simulink model "SecRwRtStArmScrnCtrl"  (R2018b)
settings: Solver=FixedStepDiscrete  StartTime=0.0  StopTime=10.0  FixedStep=0.01  RelTol=1e-3
undefined symbols (not defined in the file or in its folder): KeSMSuMdMotFinshdTm_Val, KeSMSuMdRetryTm1_Val, KeSMSuModeReqDurgTm_Val, KeSMSwSecRwRtStArmScrnEnTrigBitMask_Val
libraries: StCtrlLib x1
settings Model: Creator=sn2xws  LastModifiedBy=sn2xws
settings DataIOCC: SaveFormat=StructureWithTime
settings OptimizationCC: DefaultParameterBehavior=Inlined  EnhancedBackFolding=on  PassReuseOutputArgsAs=Individual arguments  ZeroExternalMemoryAtStartup=off  ZeroInternalMemoryAtStartup=off  OptimizeBlockOrder=speed  DifferentSizesBufferReuse=on  OptimizationCustomize=off
settings DebuggingCC: ParameterTunabilityLossMsg=error
settings ModelReferenceCC: ModelReferenceNumInstancesAllowed=Single
settings SFSimCC: MATLABDynamicMemAlloc=off
settings RTWCC: SystemTargetFile=autosar.tlc  GenCodeOnly=on  TemplateMakefile=ert_default_tmf  Description=AUTOSAR  GenerateReport=on  IncludeHyperlinkInReport=on  LaunchReport=on  GenerateTraceInfo=on  GenerateTraceReport=on  GenerateTraceReportSl=on  GenerateTraceReportSf=on  GenerateTraceReportEml=on
settings CodeAppCC: ForceParamTrailComments=on  IgnoreCustomStorageClasses=off  OperatorAnnotations=on  SimulinkDataObjDesc=on  SFDataObjDesc=on  InsertBlockDesc=on
settings STFCustomTargetCC: TargetLangStandard=C99 (ISO)  MultiwordLength=256  ParMdlRefBuildCompliant=on  CompOptLevelCompliant=on  IncludeMdlTerminateFcn=off  CombineOutputUpdateFcns=on  SuppressErrorStatus=on  ERTCustomFileBanners=on  SupportNonFinite=off  SupportComplex=off  SupportContinuousTime=off  SupportNonInlinedSFcns=off  RemoveResetFunc=on  MATLABClassNameForMDSCustomization=Simulink.SoftwareTarget.ERTCustomization  AutosarCompliant=on  UseToolchainInfoCompliant=on  LookupTableObjectStructAxisOrder=2,1,3,4,...  LUTObjectStructOrderEvenSpacing=Size,Table,Breakpoints  SystemTargetFile=autosar.tlc
settings ERTTargetCC: TargetLangStandard=C99 (ISO)  ConcurrentExecutionCompliant=off  IncludeMdlTerminateFcn=off  SuppressErrorStatus=on  SupportNonFinite=off  SupportComplex=off  ModelStepFunctionPrototypeControlCompliant=off  CPPClassGenCompliant=off  AutosarCompliant=on  LookupTableObjectStructAxisOrder=2,1,3,4,...  LUTObjectStructOrderEvenSpacing=Size,Table,Breakpoints  InlinedParameterPlacement=NonHierarchical  ERTCustomFileTemplate=example_file_process.tlc  ERTFilePackagingFormat=Compact

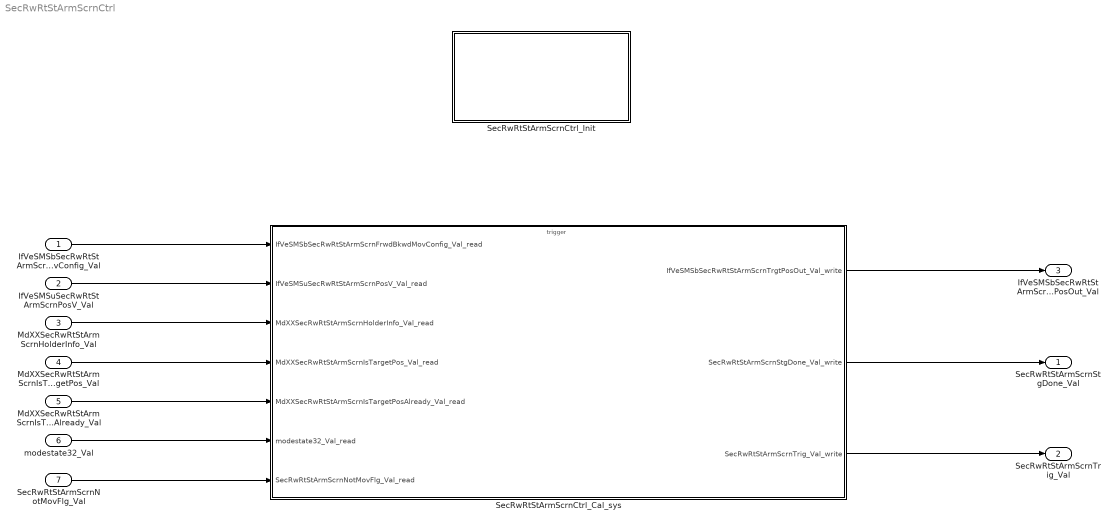
== system SecRwRtStArmScrnCtrl ==
  IfVeSMSbSecRwRtStArmScrnFrwdBkwdMovConfig_Val : Inport  OutDataTypeStr=boolean  PortDimensions=1
  IfVeSMSuSecRwRtStArmScrnPosV_Val : Inport  Port=2  OutDataTypeStr=boolean  PortDimensions=1
  MdXXSecRwRtStArmScrnHolderInfo_Val : Inport  Port=3  OutDataTypeStr=uint32  PortDimensions=1
  MdXXSecRwRtStArmScrnIsTargetPos_Val : Inport  Port=4  OutDataTypeStr=uint32  PortDimensions=1
  MdXXSecRwRtStArmScrnIsTargetPosAlready_Val : Inport  Port=5  OutDataTypeStr=uint32  PortDimensions=1
  modestate32_Val : Inport  Port=6  OutDataTypeStr=uint32  PortDimensions=1
  SecRwRtStArmScrnNotMovFlg_Val : Inport  Port=7  OutDataTypeStr=boolean  PortDimensions=1
  SecRwRtStArmScrnCtrl_Cal_sys : Subsystem
  SecRwRtStArmScrnCtrl_Init : Subsystem
  SecRwRtStArmScrnStgDone_Val : Outport  OutDataTypeStr=boolean  PortDimensions=1
  SecRwRtStArmScrnTrig_Val : Outport  Port=2  OutDataTypeStr=boolean  PortDimensions=1
  IfVeSMSbSecRwRtStArmScrnTrgtPosOut_Val : Outport  Port=3  OutDataTypeStr=boolean  PortDimensions=1
  wires:
  IfVeSMSbSecRwRtStArmScrnFrwdBkwdMovConfig_Val/1 -> SecRwRtStArmScrnCtrl_Cal_sys/1(IfVeSMSbSecRwRtStArmScrnFrwdBkwdMovConfig_Val_read)
  IfVeSMSuSecRwRtStArmScrnPosV_Val/1 -> SecRwRtStArmScrnCtrl_Cal_sys/2(IfVeSMSuSecRwRtStArmScrnPosV_Val_read)
  MdXXSecRwRtStArmScrnHolderInfo_Val/1 -> SecRwRtStArmScrnCtrl_Cal_sys/3(MdXXSecRwRtStArmScrnHolderInfo_Val_read)
  MdXXSecRwRtStArmScrnIsTargetPos_Val/1 -> SecRwRtStArmScrnCtrl_Cal_sys/4(MdXXSecRwRtStArmScrnIsTargetPos_Val_read)
  MdXXSecRwRtStArmScrnIsTargetPosAlready_Val/1 -> SecRwRtStArmScrnCtrl_Cal_sys/5(MdXXSecRwRtStArmScrnIsTargetPosAlready_Val_read)
  modestate32_Val/1 -> SecRwRtStArmScrnCtrl_Cal_sys/6(modestate32_Val_read)
  SecRwRtStArmScrnNotMovFlg_Val/1 -> SecRwRtStArmScrnCtrl_Cal_sys/7(SecRwRtStArmScrnNotMovFlg_Val_read)
  SecRwRtStArmScrnCtrl_Cal_sys/1(IfVeSMSbSecRwRtStArmScrnTrgtPosOut_Val_write) -> IfVeSMSbSecRwRtStArmScrnTrgtPosOut_Val/1
  SecRwRtStArmScrnCtrl_Cal_sys/2(SecRwRtStArmScrnStgDone_Val_write) -> SecRwRtStArmScrnStgDone_Val/1
  SecRwRtStArmScrnCtrl_Cal_sys/3(SecRwRtStArmScrnTrig_Val_write) -> SecRwRtStArmScrnTrig_Val/1

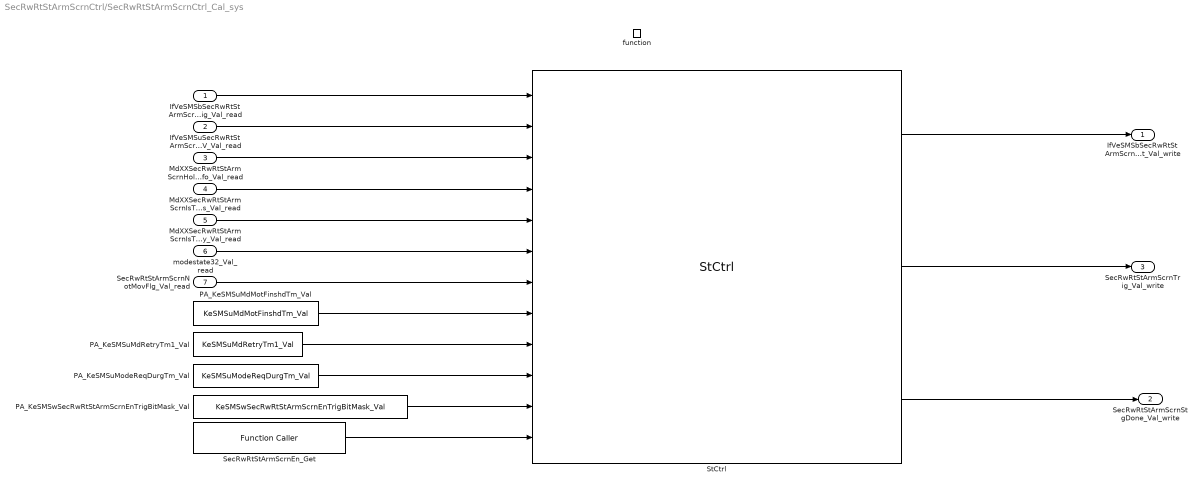
== system SecRwRtStArmScrnCtrl/SecRwRtStArmScrnCtrl_Cal_sys ==
  IfVeSMSbSecRwRtStArmScrnFrwdBkwdMovConfig_Val_read : Inport
  IfVeSMSuSecRwRtStArmScrnPosV_Val_read : Inport  Port=2
  MdXXSecRwRtStArmScrnHolderInfo_Val_read : Inport  Port=3
  MdXXSecRwRtStArmScrnIsTargetPos_Val_read : Inport  Port=4
  MdXXSecRwRtStArmScrnIsTargetPosAlready_Val_read : Inport  Port=5
  modestate32_Val_read : Inport  Port=6
  SecRwRtStArmScrnNotMovFlg_Val_read : Inport  Port=7
  function : TriggerPort  TriggerType=function-call  IsSimulinkFunction=on  FunctionName=SecRwRtStArmScrnCtrl_Cal  VariantControl=(inherit)
  PA_KeSMSuMdMotFinshdTm_Val : Constant  Value=KeSMSuMdMotFinshdTm_Val
  PA_KeSMSuMdRetryTm1_Val : Constant  Value=KeSMSuMdRetryTm1_Val
  PA_KeSMSuModeReqDurgTm_Val : Constant  Value=KeSMSuModeReqDurgTm_Val
  PA_KeSMSwSecRwRtStArmScrnEnTrigBitMask_Val : Constant  Value=KeSMSwSecRwRtStArmScrnEnTrigBitMask_Val
  SecRwRtStArmScrnEn_Get : FunctionCaller  FunctionPrototype=data = SecRwRtStArmScrnEn_Get()  OutputArgumentSpecifications=uint32(1)
  StCtrl : StCtrlLib/StCtrl  SystemSampleTime=-1
  IfVeSMSbSecRwRtStArmScrnTrgtPosOut_Val_write : Outport
      settings: EnsureOutportIsVirtual=on
  SecRwRtStArmScrnStgDone_Val_write : Outport  Port=2
      settings: EnsureOutportIsVirtual=on
  SecRwRtStArmScrnTrig_Val_write : Outport  Port=3
      settings: EnsureOutportIsVirtual=on
  wires:
  StCtrl/3 -> SecRwRtStArmScrnStgDone_Val_write/1
  StCtrl/1 -> IfVeSMSbSecRwRtStArmScrnTrgtPosOut_Val_write/1
  StCtrl/2 -> SecRwRtStArmScrnTrig_Val_write/1
  PA_KeSMSwSecRwRtStArmScrnEnTrigBitMask_Val/1 -> StCtrl/11
  SecRwRtStArmScrnEn_Get/1 -> StCtrl/12
  PA_KeSMSuModeReqDurgTm_Val/1 -> StCtrl/10
  PA_KeSMSuMdMotFinshdTm_Val/1 -> StCtrl/8
  PA_KeSMSuMdRetryTm1_Val/1 -> StCtrl/9
  MdXXSecRwRtStArmScrnIsTargetPos_Val_read/1 -> StCtrl/4
  MdXXSecRwRtStArmScrnIsTargetPosAlready_Val_read/1 -> StCtrl/5
  IfVeSMSbSecRwRtStArmScrnFrwdBkwdMovConfig_Val_read/1 -> StCtrl/1
  IfVeSMSuSecRwRtStArmScrnPosV_Val_read/1 -> StCtrl/2
  MdXXSecRwRtStArmScrnHolderInfo_Val_read/1 -> StCtrl/3
  modestate32_Val_read/1 -> StCtrl/6
  SecRwRtStArmScrnNotMovFlg_Val_read/1 -> StCtrl/7

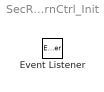
== system SecRwRtStArmScrnCtrl/SecRwRtStArmScrnCtrl_Init ==
  Event Listener : EventListener  EventName=reset
